simulink model "Darko"  (R2026a)
settings: Solver=VariableStepAuto
values from neighbouring files (symbols this model uses):
  delta_inertia = 0    [DARKO_MAIN.m]    (also in DARKO_MAIN_long.m; check_Darko_long.m)
  delta_mass = 0    [DARKO_MAIN.m]    (also in DARKO_MAIN_long.m; check_Darko_long.m)
  delta_phi_coef = 0.0    (= 0)    [DARKO_MAIN.m]    (also in DARKO_MAIN_long.m; check_Darko_long.m)
  time_var_param = 13500    [DARKO_MAIN.m]    (also in DARKO_MAIN_long.m = inf; check_Darko_long.m = inf)
  Ts = 1/500    (= 0.002)    [DARKO_MAIN.m]    (also in DARKO_MAIN_long.m; check_Darko_long.m)
  xj0 = [vb; wb; q]    [DARKO_MAIN.m]    (also in DARKO_MAIN_long.m = xts(:, trim_sol); check_Darko_long.m = xt)
libraries: sharedtransform x1
settings Model: Creator=devinbellll  LastModifiedBy=devinbellll

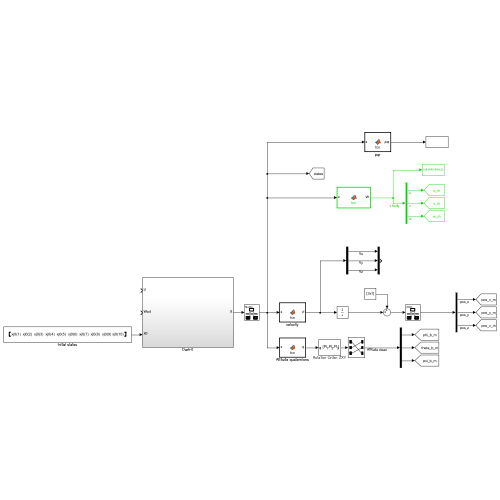
[thumbnail: Simulink's stored preview of the top-level diagram]
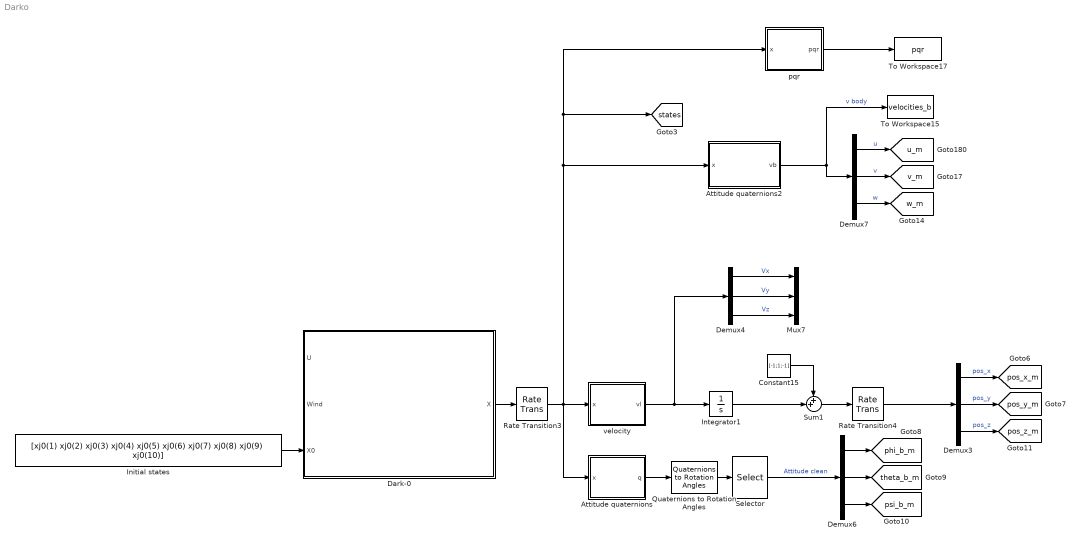
== system Darko ==
  Attitude quaternions : MATLAB Function  TreatAsAtomicUnit=on
  Attitude quaternions2 : MATLAB Function  TreatAsAtomicUnit=on
  Constant15 : Constant  Value=[-1;1;-1]  SampleTime=Ts
  Dark-0 : Subsystem
  Demux{3..4,6..7} (4 alike) : Demux  Outputs=3
  Initial states : Constant  Value=[xj0(1) xj0(2) xj0(3) xj0(4) xj0(5) xj0(6) xj0(7) xj0(8) xj0(9) xj0(10)]  SampleTime=Ts
  Integrator1 : Integrator  InitialCondition=[1;-1;1.20]
  Mux7 : Mux  Inputs=3
  Quaternions to Rotation Angles : sharedtransform/Quaternions to Rotation Angles  rotationOrder=ZXY  aMode=aMode
  Rate Transition3 : RateTransition  OutPortSampleTime=Ts
  Rate Transition4 : RateTransition  OutPortSampleTime=Ts
  Selector : Selector  InputPortWidth=3  IndexOptions=Index vector (dialog)  Indices=[2 3 1]  OutputSizes=1
  Sum1 : Sum  Inputs=++|
  To Workspace15 : ToWorkspace  VariableName=velocities_b  SampleTime=Ts
  To Workspace17 : ToWorkspace  VariableName=pqr  SampleTime=Ts
  pqr : MATLAB Function  TreatAsAtomicUnit=on
  velocity : MATLAB Function  TreatAsAtomicUnit=on
  tag scope: phi_b_m=global, pos_x_m=global, pos_y_m=global, pos_z_m=global, psi_b_m=global, states=global, theta_b_m=global, u_m=global, v_m=global, w_m=global
  wires:
  Demux7/2 -> [v_m]  "v"
  Demux3/3 -> [pos_z_m]  "pos_z"
  pqr/1(pqr) -> To Workspace17/1
  Demux4/1 -> Mux7/1  "Vx"
  Demux6/2 -> [theta_b_m]
  Demux3/2 -> [pos_y_m]  "pos_y"
  Constant15/1 -> Sum1/1
  Demux3/1 -> [pos_x_m]  "pos_x"
  Integrator1/1 -> Sum1/2
  Demux7/1 -> [u_m]  "u"
  Demux4/2 -> Mux7/2  "Vy"
  Demux6/3 -> [psi_b_m]
  Rate Transition4/1 -> Demux3/1
  Demux6/1 -> [phi_b_m]
  Sum1/1 -> Rate Transition4/1
  velocity/1(vl) -> Integrator1/1, Demux4/1
  Quaternions to Rotation Angles/1 -> Selector/1
  Attitude quaternions/1(q) -> Quaternions to Rotation Angles/1
  Demux4/3 -> Mux7/3  "Vz"
  Attitude quaternions2/1(vb) -> Demux7/1, To Workspace15/1  "v body"
  Demux7/3 -> [w_m]  "w"
  Initial states/1 -> Dark-0/3(X0)
  Rate Transition3/1 -> Attitude quaternions/1(x), velocity/1(x), pqr/1(x), [states], Attitude quaternions2/1(x)
  Dark-0/1(X) -> Rate Transition3/1
  Selector/1 -> Demux6/1  "Attitude clean"

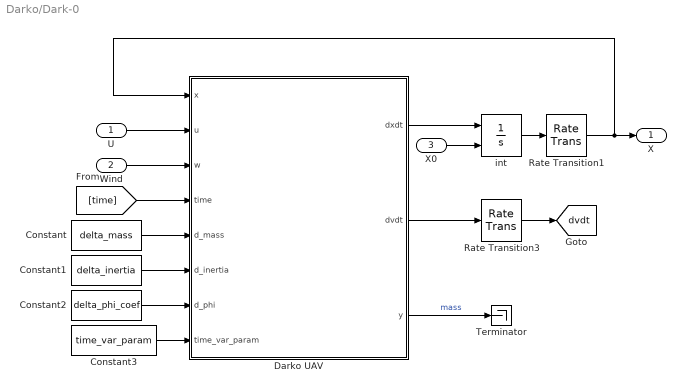
== system Darko/Dark-0 ==
  U : Inport
  Wind : Inport  Port=2
  X0 : Inport  Port=3
  Constant : Constant  Value=delta_mass  SampleTime=Ts
  Constant1 : Constant  Value=delta_inertia  SampleTime=Ts
  Constant2 : Constant  Value=delta_phi_coef  SampleTime=Ts
  Constant3 : Constant  Value=time_var_param  SampleTime=Ts
  Darko UAV : MATLAB Function  TreatAsAtomicUnit=on
  Rate Transition1 : RateTransition  OutPortSampleTime=Ts
  Rate Transition3 : RateTransition  OutPortSampleTime=Ts
  Terminator : Terminator
  int : Integrator  InitialConditionSource=external
  X : Outport  VectorParamsAs1DForOutWhenUnconnected=off
  tag scope: dvdt=global
  wires:
  U/1 -> Darko UAV/2(u)
  Darko UAV/1(dxdt) -> int/1
  Wind/1 -> Darko UAV/3(w)
  X0/1 -> int/2
  Darko UAV/2(dvdt) -> Rate Transition3/1
  Rate Transition3/1 -> [dvdt]
  int/1 -> Rate Transition1/1
  Rate Transition1/1 -> X/1, Darko UAV/1(x)
  [time] -> Darko UAV/4(time)
  Constant/1 -> Darko UAV/5(d_mass)
  Constant2/1 -> Darko UAV/7(d_phi)
  Constant1/1 -> Darko UAV/6(d_inertia)
  Darko UAV/3(y) -> Terminator/1  "mass"
  Constant3/1 -> Darko UAV/8(time_var_param)

== matlab function Darko/Attitude quaternions ==
  data: x input; q output
function q  = fcn(x)
%#codegen

%% quaternion computation
q = x(7:10);

== matlab function Darko/Dark-0/Darko UAV ==
  data: x input; u input; dxdt output; w input; dvdt output; time input; d_mass input; d_inertia input; d_phi input; time_var_param input; y output
function [dxdt, dvdt,y] = fcn(x, u, w, time, d_mass, d_inertia, d_phi, time_var_param)
%#codegen

drone = generateDarko();
y = drone.MASS;

% if(time > time_var_param*1000)
%     drone.MASS    = drone.MASS - d_mass*drone.MASS;
%     drone.INERTIA = drone.INERTIA - d_inertia*drone.INERTIA;
%     drone.PHI     = drone.PHI - d_phi*drone.PHI;
%     y = drone.MASS;
% end
if(time > -1)
    drone.MASS    = drone.MASS + 0.6*drone.MASS;
    drone.INERTIA = drone.INERTIA + 0.6*drone.INERTIA;
    drone.PHI     = drone.PHI + 0.6*drone.PHI;
    drone.CHORD   = drone.CHORD + 0.6*drone.CHORD;
    drone.WINGSPAN = drone.WINGSPAN + 0.6*drone.WINGSPAN;
    y = drone.MASS;
end
dxdt = sysEqt(x, u, w, drone);
dvdt = dxdt(1:3);

== matlab function Darko/velocity ==
  data: x input; vl output
function vl  = fcn(x)
%#codegen

vl = x(1:3);
%q  = x(7:10,1);
%D = q2dcm(q');

%vb = D*vl;
%vb(3) = -vb(3); % NED coordinate

%vl(3) = -x(3);

== matlab function Darko/Attitude quaternions2 ==
  data: x input; vb output
function vb   = fcn(x)
%#codegen

vl = x(1:3);
%% quaternion and DCM computation
q  = x(7:10,1);
D = q2dcm(q');


%% speed in body-frame
vb = D*vl;

== matlab function Darko/pqr ==
  data: x input; pqr output
function pqr  = fcn(x)
%#codegen

pqr = x(4:6);
